simulink model "Sim35"  (R2019a)
settings: Solver=FixedStepAuto  StartTime=0.0  StopTime=10.0  FixedStep=0.0001  RelTol=1e-3
settings Model: Creator=fbleo  LastModifiedBy=fbleo

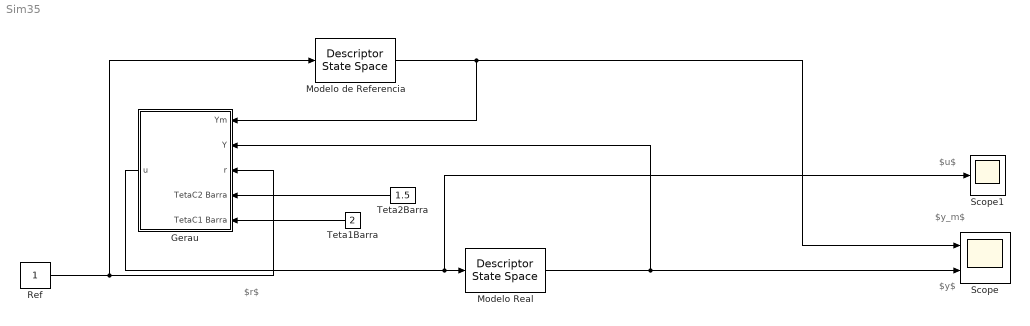
== system Sim35 ==
  note: $u$
  note: $y$
  note: $y_m$
  note: $r$
  Gerau : Subsystem
  Modelo Real : DescriptorStateSpace  A=-1  B=2  D=0  InitialCondition=0.5
  Modelo de Referencia : DescriptorStateSpace  A=-3  B=3  D=0  InitialCondition=0
  Ref : Constant
  Scope : Scope  NumInputPorts=2
  Scope1 : Scope
  Teta1Barra : Constant  Value=2
  Teta2Barra : Constant  Value=1.5
  wires:
  Teta2Barra/1 -> Gerau/4(TetaC2 Barra)
  Ref/1 -> Modelo de Referencia/1, Gerau/3(r)
  Gerau/1(u) -> Scope1/1, Modelo Real/1
  Modelo Real/1 -> Gerau/2(Y), Scope/2
  Modelo de Referencia/1 -> Scope/1, Gerau/1(Ym)
  Teta1Barra/1 -> Gerau/5(TetaC1 Barra)

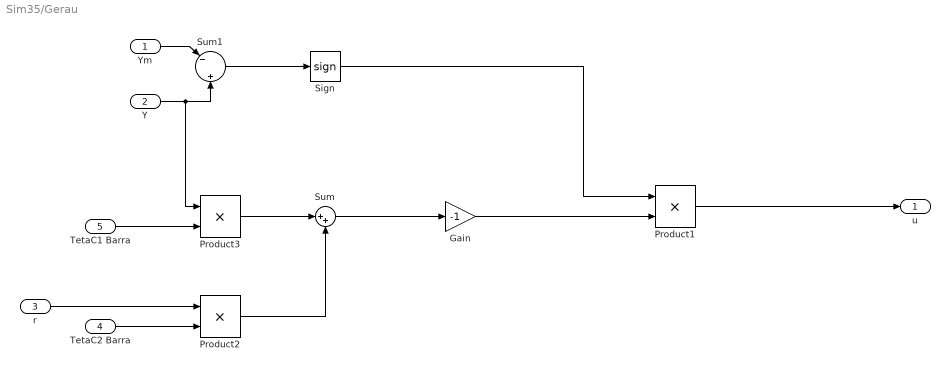
== system Sim35/Gerau ==
  Ym : Inport
  Y : Inport  Port=2
  r : Inport  Port=3
  TetaC2 Barra : Inport  Port=4
  TetaC1 Barra : Inport  Port=5
  Gain : Gain  Gain=-1
  Product1 : Product
  Product2 : Product
  Product3 : Product
  Sign : Signum
  Sum : Sum  Inputs=|++
  Sum1 : Sum  Inputs=|-||+
  u : Outport
  wires:
  Ym/1 -> Sum1/1
  Y/1 -> Product3/1, Sum1/2
  Sum1/1 -> Sign/1
  r/1 -> Product2/1
  Product1/1 -> u/1
  Sign/1 -> Product1/1
  TetaC2 Barra/1 -> Product2/2
  TetaC1 Barra/1 -> Product3/2
  Product3/1 -> Sum/1
  Product2/1 -> Sum/2
  Sum/1 -> Gain/1
  Gain/1 -> Product1/2
